simulink model "gravityGradTorqueISS_sl"  (R2024b)
settings: Solver=VariableStepAuto  StartTime=0.0  StopTime=10.0  RelTol=1e-3
settings Model: Creator=gilbu
settings RTWCC: GPUComputeCapability=3.5

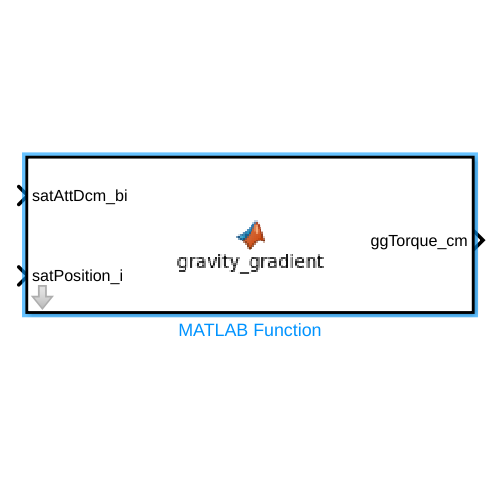
[thumbnail: Simulink's stored preview of the top-level diagram]
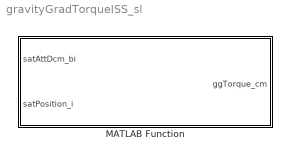
== system gravityGradTorqueISS_sl ==
  MATLAB Function : MATLAB Function  TreatAsAtomicUnit=on

== matlab function gravityGradTorqueISS_sl/MATLAB Function ==
  data: ggTorque_cm output; satAttDcm_bi input; satPosition_i input
% Author: Thomas Holzman
function ggTorque_cm = gravity_gradient ( ...
    satAttDcm_bi,satPosition_i)...%inputs)
%-------------------------------------------------------------------------------
%Torque Calculations

r_b= satAttDcm_bi*satPosition_i; % [m]
mu = 3.98e14; %m^3/s^2

Jb = [70942261 3512761 3543989;
      3512761 59070966 -2768801;   %kg*m^2
      3543989 -2768801 123909888];

nr = norm (r_b);
db= -r_b/nr;

ggTorque_cm = 3*mu/nr^3*cross(db, Jb*db); %N*m
